simulink model "Q2_sim_control"  (Simulink 7.0)
settings: Solver=ode45  StartTime=0.0  StopTime=10  RelTol=1e-3
libraries: simulink_extras x1
settings Model: Creator=Fares Hesham  LastModifiedBy=Fares Hesham

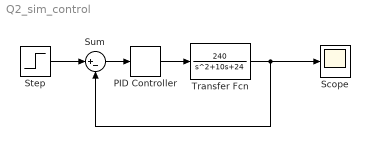
== system Q2_sim_control ==
  PID Controller : simulink_extras/Additional Linear/PID Controller  SystemSampleTime=-1  P=1  I=1  D=1
  Scope : Scope
  Step : Step  Time=0  SampleTime=10
  Sum : Sum  Inputs=|+-  OutDataType=sfix(16)  OutScaling=2^0
  Transfer Fcn : TransferFcn  Numerator=[240]  Denominator=[1 10 24]
  wires:
  Transfer Fcn/1 -> Sum/2, Scope/1
  Step/1 -> Sum/1
  Sum/1 -> PID Controller/1
  PID Controller/1 -> Transfer Fcn/1
